simulink model "sdnf"  (Simulink 7.4)
settings: Solver=ode45  StartTime=0.0  StopTime=10.0  RelTol=1e-3
settings Model: Creator=autologin  LastModifiedBy=autologin

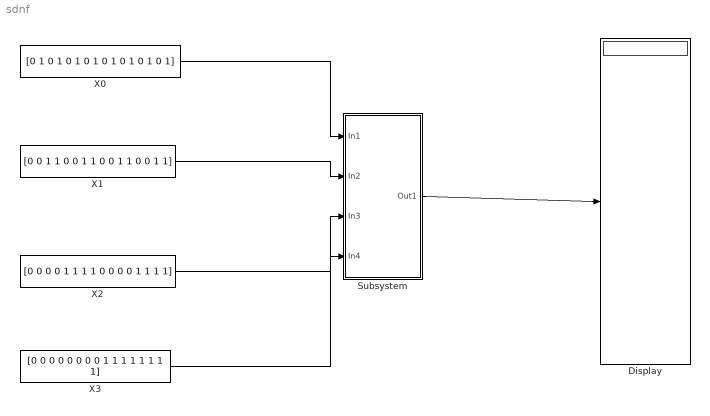
== system sdnf ==
  Display : Display
  Subsystem : Subsystem
  X0 : Constant  Value=[0 1 0 1 0 1 0 1 0 1 0 1 0 1 0 1]  OutDataType=fixdt(1, 16)  OutScaling=2^0
  X1 : Constant  Value=[0 0 1 1 0 0 1 1 0 0 1 1 0 0 1 1]  OutDataType=fixdt(1, 16)  OutScaling=2^0
  X2 : Constant  Value=[0 0 0 0 1 1 1 1 0 0 0 0 1 1 1 1]  OutDataType=fixdt(1, 16)  OutScaling=2^0
  X3 : Constant  Value=[0 0 0 0 0 0 0 0 1 1 1 1 1 1 1 1]  OutDataType=fixdt(1, 16)  OutScaling=2^0
  wires:
  Subsystem/1(Out1) -> Display/1
  X0/1 -> Subsystem/1(In1)
  X2/1 -> Subsystem/3(In3)
  X1/1 -> Subsystem/2(In2)
  X3/1 -> Subsystem/4(In4)

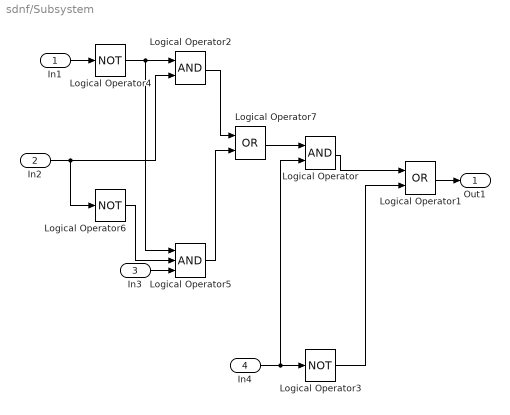
== system sdnf/Subsystem ==
  In1 : Inport
  In2 : Inport  Port=2
  In3 : Inport  Port=3
  In4 : Inport  Port=4
  Logical Operator : Logic  AllPortsSameDT=off  OutDataTypeMode=boolean  LogicDataType=fixdt(0, 8)  OutDataTypeStr=boolean
  Logical Operator1 : Logic  Operator=OR  AllPortsSameDT=off  OutDataTypeMode=boolean  LogicDataType=fixdt(0, 8)  OutDataTypeStr=boolean
  Logical Operator2 : Logic  AllPortsSameDT=off  OutDataTypeMode=boolean  LogicDataType=fixdt(0, 8)  OutDataTypeStr=boolean
  Logical Operator3 : Logic  Operator=NOT  Inputs=3  AllPortsSameDT=off  OutDataTypeMode=boolean  LogicDataType=fixdt(0, 8)  OutDataTypeStr=boolean
  Logical Operator4 : Logic  Operator=NOT  Inputs=3  AllPortsSameDT=off  OutDataTypeMode=boolean  LogicDataType=fixdt(0, 8)  OutDataTypeStr=boolean
  Logical Operator5 : Logic  Inputs=3  AllPortsSameDT=off  OutDataTypeMode=boolean  LogicDataType=fixdt(0, 8)  OutDataTypeStr=boolean
  Logical Operator6 : Logic  Operator=NOT  Inputs=3  AllPortsSameDT=off  OutDataTypeMode=boolean  LogicDataType=fixdt(0, 8)  OutDataTypeStr=boolean
  Logical Operator7 : Logic  Operator=OR  AllPortsSameDT=off  OutDataTypeMode=boolean  LogicDataType=fixdt(0, 8)  OutDataTypeStr=boolean
  Out1 : Outport
  wires:
  In4/1 -> Logical Operator/2, Logical Operator3/1
  Logical Operator3/1 -> Logical Operator1/2
  In2/1 -> Logical Operator2/2, Logical Operator6/1
  Logical Operator/1 -> Logical Operator1/1
  Logical Operator4/1 -> Logical Operator2/1, Logical Operator5/1
  Logical Operator6/1 -> Logical Operator5/2
  Logical Operator7/1 -> Logical Operator/1
  Logical Operator2/1 -> Logical Operator7/1
  Logical Operator5/1 -> Logical Operator7/2
  In1/1 -> Logical Operator4/1
  Logical Operator1/1 -> Out1/1
  In3/1 -> Logical Operator5/3
